simulink model "adaptive_multi_task"  (R2023b)
settings: Solver=VariableStepAuto  StartTime=0.0  StopTime=11  FixedStep=0.001
libraries: robotmaniplib x1, simulink_extras x1
settings Model: Creator=ACL_2024N02  LastModifiedBy=ACL_2024N02

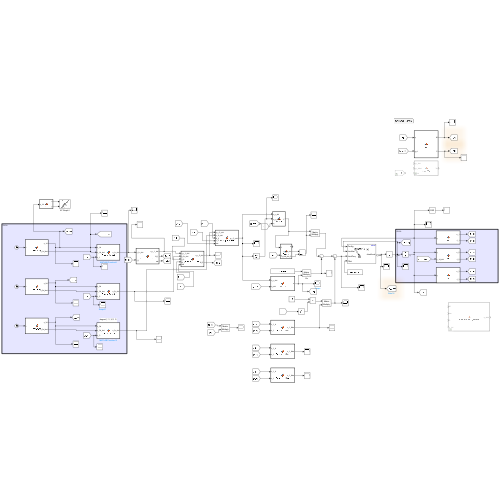
[thumbnail: Simulink's stored preview of the top-level diagram]
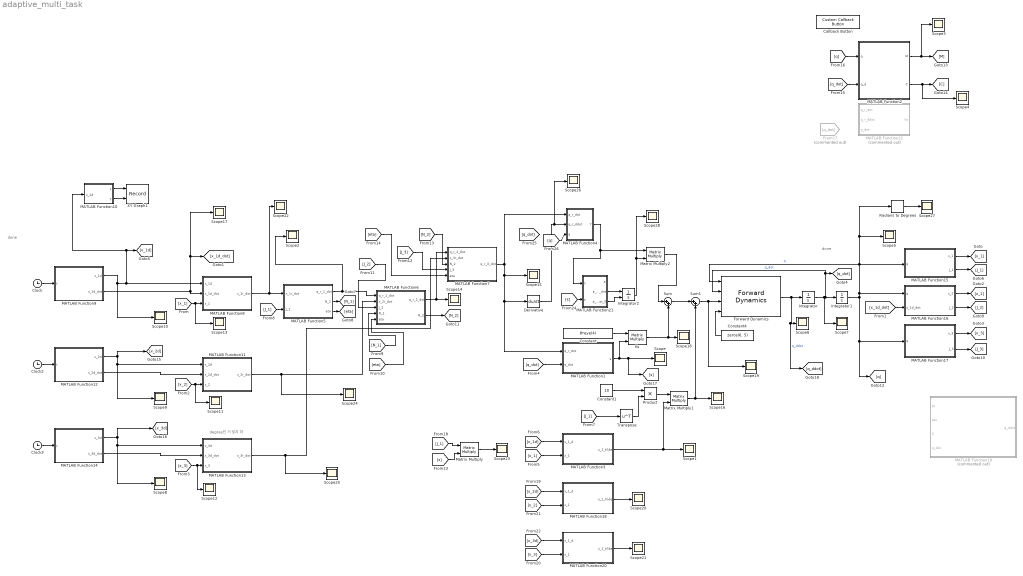
== system adaptive_multi_task ==
  note: done
  note: degree인 거 잊지 마
  note: done
  Callback Button : CustomCallbackButton  Configuration="{\"components\":[{\"name\":\"BackgroundImageComponent\",\"settings\":{\"image\":{\"size\":[0,0],\"src\":\"default\",\"srcOrientation\":\"Right\"},\"position\":[0,0,1,1]}},{\"name\":\"ButtonStateComponent\",\"settings\":{\"buttonType\":\"momentary\",\"clickFcn\":\"%% Robot kinematics setup \\n\\nrobot = rigidBodyTree;\\n\\n% 링크 생성\\nlink0 = rigidBody('link0');\\nlink1 = rigidBody('link1');\\nlink2 = rigidBody('link2');\\nlink3 = rigidBody('link3');\\nlink4 = rigidBody('link4');\\n\\n% 조인트 생성\\njoint0 = rigidBodyJoint('joint0','revolute');\\njoint1 = rigidBodyJoint('joint1','revolute');\\njoint2 = rigidBodyJoint('joint2','revolute');\\njoint3 = rigidBodyJoint('joint3','revolute');\\njoint4 = rigidBodyJoint('joint4','fixed');\\n\\n% 링크 길이 정의\\nlink_lengths = [0.5 0.4 0.35 0.2];\\n\\n% 각 조인트의 상대 위치 지정 (이전 링크 기준 x축 방향으로 이동)\\nsetFixedTransform(joint0, trvec2tform([0, 0, 0]));            % base 위치\\nsetFixedTransform(joint1, trvec2tform([link_lengths(1), 0, 0]));\\nsetFixedTransform(joint2, trvec2tform([link_lengths(2), 0, 0]));\\nsetFixedTransform(joint3, trvec2tform([link_lengths(3), 0, 0]));\\nsetFixedTransform(joint4, trvec2tform([link_lengths(4), 0, 0]));\\n\\n% 조인트를 링크에 부착\\nlink0.Joint = joint0;\\nlink1.Joint = joint1;\\nlink2.Joint = joint2;\\nlink3.Joint = joint3;\\nlink4.Joint = joint4;   \\n\\n% 링크를 트리에 추가\\naddBody(robot, link0, 'base');\\naddBody(robot, link1, 'link0');\\naddBody(robot, link2, 'link1');\\naddBody(robot, link3, 'link2');\\naddBody(robot, link4, 'link3');\\n\\n% 로봇 정보 확인\\nshowdetails(robot);\",\"onValue\":1,\"position\":[0,0,1,1],\"pressDelay\":\"500\",\"pressFcn\":\"\",\"repeatInterval\":\"0\",\"states\":[{\"horizontalAlignment\":\"center\",\"image\":{\"position\":[0,0,1,1],\"size\":[1,1],\"src\":\"default\",\"srcOrientation\":\"Right\"},\"label\":{\"color\":[0.01176470588,0.01176470588,0.01176470588,1],\"icon\":{\"size\":[0,0],\"src\":\"default\",\"srcOrientation\":\"Right\"},\"iconPlacement\":\"left\",\"opacity\":1,\"show\":true,\"text\":{\"content\":\"Callback Button\",\"font\":\"Helvetica\",\"fontSize\":9.600000000000001}},\"labelOffset\":[0,0],\"verticalAlignment\":\"middle\"},{\"horizontalAlignment\":\"center\",\"image\":{\"position\":[0,0,1,1],\"size\":[1,1],\"src\":\"default\",\"srcOrientation\":\"Right\"},\"label\":{\"color\":[0.01176470588,0.01176470588,0.01176470588,1],\"icon\":{\"size\":[0,0],\"src\":\"default\",\"srcOrientation\":\"Right\"},\"iconPlacement\":\"left\",\"opacity\":1,\"show\":true,\"text\":{\"content\":\"Callback Button\",\"font\":\"Helvetica\",\"fontSize\":9.600000000000001}},\"labelOffset\":[0,0],\"verticalAlignment\":\"middle\"},{\"horizontalAlignment\":\"center\",\"image\":{\"position\":[0,0,1,1],\"size\":[1,1],\"src\":\"default\",\"srcOrientation\":\"Right\"},\"label\":{\"color\":[0.01176470588,0.01176470588,0.01176470588,1],\"icon\":{\"size\":[0,0],\"src\":\"default\",\"srcOrientation\":\"Right\"},\"iconPlacement\":\"left\",\"opacity\":1,\"show\":true,\"text\":{\"content\":\"Callback Button\",\"font\":\"Helvetica\",\"fontSize\":9.600000000000001}},\"labelOffset\":[0,0],\"verticalAlignment\":\"middle\"},{\"horizontalAlignment\":\"center\",\"image\":{\"position\":[0,0,1,1],\"size\":[1,1],\"src\":\"default\",\"srcOrientation\":\"Right\"},\"label\":{\"color\":[0.01176470588,0.01176470588,0.01176470588,1],\"icon\":{\"size\":[0,0],\"src\":\"default\",\"srcOrientation\":\"Right\"},\"iconPlacement\":\"left\",\"opacity\":1,\"show\":true,\"text\":{\"content\":\"Callback Button\",\"font\":\"Helvetica\",\"fontSize\":9.600000000000001}},\"labelOffset\":[0,0],\"verticalAlignment\":\"middle\"}]}},{\"name\":\"ForegroundImageComponent\",\"settings\":{\"image\":{\"size\":[0,0],\"src\":\"default\",\"srcOrientation\":\"Right\"},\"isForeground\":1,\"position\":[0,0,1,1]}}],\"settings\":{\"BindingType\":\"standalone\",\"backgroundColor\":[244,244,244,1],\"backgroundOffset\":0.2,\"backgroundOpacity\":1,\"fixedAspectRatio\":\"off\",\"foregroundColor\":[0.01176470588,0.01176470588,0.01176470588,1],\"migratedFromLegacy\":true,\"useBackgroundColor\":true,\"variant\":\"callback\",\"version\":\"R2023a\"},\"type\":\"Button\"}"  CustomBackgroundColor="{\"color\":[0.9568627451,0.9568627451,0.9568627451],\"show\":true}"
  Clock : Clock
  Clock2 : Clock
  Clock3 : Clock
  Constant : Constant  Value=8*eye(4)
  Constant1 : Constant  Value=10
  Constant4 : Constant  Value=zeros(6, 5)
  Derivative : Derivative
  Forward Dynamics : robotmaniplib/Forward Dynamics  RigidBodyTree=robot  SimulateUsing=Code generation
  From17 : From  Commented=on  GotoTag=q_dot
  Integrator : Integrator  UpperSaturationLimit=pi  LowerSaturationLimit=-pi
  Integrator1 : Integrator  InitialCondition=[0.8727; 1.7; -1.6; 0.85]  UpperSaturationLimit=pi  LowerSaturationLimit=-pi
  Integrator2 : Integrator  InitialConditionSource=external
  Ks : Product  Multiplication=Matrix(*)
  MATLAB Function1 : MATLAB Function  TreatAsAtomicUnit=on
  MATLAB Function10 : MATLAB Function  TreatAsAtomicUnit=on
  MATLAB Function11 : MATLAB Function  TreatAsAtomicUnit=on
  MATLAB Function12 : MATLAB Function  TreatAsAtomicUnit=on
  MATLAB Function13 : MATLAB Function  TreatAsAtomicUnit=on
  MATLAB Function14 : MATLAB Function  TreatAsAtomicUnit=on
  MATLAB Function15 : MATLAB Function  TreatAsAtomicUnit=on
  MATLAB Function16 : MATLAB Function  TreatAsAtomicUnit=on
  MATLAB Function17 : MATLAB Function  TreatAsAtomicUnit=on
  MATLAB Function18 : MATLAB Function  TreatAsAtomicUnit=on
  MATLAB Function19 : MATLAB Function  Commented=on  TreatAsAtomicUnit=on
  MATLAB Function2 : MATLAB Function  TreatAsAtomicUnit=on
  MATLAB Function20 : MATLAB Function  TreatAsAtomicUnit=on
  MATLAB Function21 : MATLAB Function  TreatAsAtomicUnit=on
  MATLAB Function22 : MATLAB Function  Commented=on  TreatAsAtomicUnit=on
  MATLAB Function3 : MATLAB Function  TreatAsAtomicUnit=on
  MATLAB Function4 : MATLAB Function  TreatAsAtomicUnit=on
  MATLAB Function5 : MATLAB Function  TreatAsAtomicUnit=on
  MATLAB Function6 : MATLAB Function  TreatAsAtomicUnit=on
  MATLAB Function7 : MATLAB Function  TreatAsAtomicUnit=on
  MATLAB Function8 : MATLAB Function  TreatAsAtomicUnit=on
  MATLAB Function9 : MATLAB Function  TreatAsAtomicUnit=on
  Matrix Multiply : Product  Multiplication=Matrix(*)
  Matrix Multiply1 : Product  Multiplication=Matrix(*)
  Matrix Multiply2 : Product  Multiplication=Matrix(*)
  Product : Product
  Radians to Degrees : simulink_extras/Transformations/Radians to Degrees
  Scope{,1..28} (29 alike) : Scope
  Sum : Sum  Inputs=|++
  Sum1 : Sum  Inputs=|++
  Transpose : Math  Operator=transpose
  XY Graph1 : Record  FileSettingsInternal="{\"entries\":[{\"content\":{\"excelSettings\":{\"content\":{},\"type\":\"Streamout.ExcelSettings\"}},\"type\":\"Streamout.FileSettingStorage\",\"uuid\":\"\"}],\"packageUris\":[\"http:\\/\\/schema.mathworks.com\\/mf0\\/streamout_blocks\\/R2020a\"],\"version\":\"1.0\"}"  Layout=[1 1]  SignalsInternal="{\"entries\":[{\"content\":{\"signals\":[{\"content\":{\"blockPath\":[],\"dimensions\":[1],\"domain\":\"\",\"lineColor\":\"#a2142f\",\"plots\":[ 1 ],\"port\":1,\"sid\":[\"\"],\"signalID\":1,\"signalName\":\"MATLAB Function10:1\"},\"type\":\"RecordBlkView.Signal\",\"uuid\":\"\"},{\"content\":{\"blockPath\":[],\"dimensions\":[1],\"domain\":\"\",\"lineColor\":\"#139fff\",\"plots\":[ 1 ],\"port\":2,\"sid\":[\"\"],\"signalID\":2,\"signalName\":\"MATLAB Function10:2\"},\"type\":\"RecordBlkView.Signal\",\"uuid\":\"\"}]},\"type\":\"RecordBlkView.InputSignals\",\"uuid\":\"\"}],\"packageUris\":[\"http:\\/\\/schema.mathworks.com\\/mf0\\/streamout_blocks\\/R2020a\"],\"version\":\"1.0\"}"  VisualizationBindings="{\"xyplotplugin\":{\"info\":[{\"series\":[{\"bindingParametersList\":[{\"parameter\":\"X-Axis\",\"signalID\":1,\"signalName\":\"MATLAB Function10:1\"},{\"parameter\":\"Y-Axis\",\"signalID\":2,\"signalName\":\"MATLAB Function10:2\"}],\"seriesID\":0}],\"subplotID\":1}]}}"  CompatibilityTag=XY
  wires:
  Constant/1 -> Ks/1
  MATLAB Function1/1(s) -> Ks/2, Scope/1, [s]
  [J_1] -> Transpose/1
  Constant1/1 -> Product/1
  Product/1 -> Matrix Multiply1/1
  MATLAB Function3/1(x_1_tilde) -> Scope1/1, Matrix Multiply1/2
  Ks/1 -> Scope18/1, Sum/2
  Sum/1 -> Sum1/1
  Matrix Multiply1/1 -> Sum1/2, Scope16/1
  Sum1/1 -> Scope19/1, Forward Dynamics/3
  Constant4/1 -> Forward Dynamics/4
  Forward Dynamics/1 -> [q_ddot], Scope6/1, Integrator/1  "q_ddot"
  Integrator/1 -> Integrator1/1, Forward Dynamics/2, [q_dot], Scope7/1  "q_dot"
  Integrator1/1 -> Forward Dynamics/1, Radians to Degrees/1, Scope5/1, MATLAB Function15/1(q), MATLAB Function16/1(q), [q], MATLAB Function17/1(q)  "q"
  MATLAB Function5/1(q_r_1_dot) -> Scope2/1, MATLAB Function6/1(q_r_1_dot)
  MATLAB Function6/1(q_r_2_dot) -> Scope14/1, MATLAB Function7/1(q_r_2_dot)
  MATLAB Function7/1(q_r_3_dot) -> Derivative/1, MATLAB Function1/1(q_r_dot), Scope15/1, MATLAB Function4/1(q_r_dot)
  MATLAB Function9/1(x_1d) -> Scope10/1, MATLAB Function8/1(x_1d), MATLAB Function10/1(x_1d), [x_1d]
  MATLAB Function9/2(x_1d_dot) -> MATLAB Function8/2(x_1d_dot), [x_1d_dot], Scope17/1
  Clock/1 -> MATLAB Function9/1(t)
  MATLAB Function8/1(x_1r_dot) -> Scope22/1, MATLAB Function5/1(x_1r_dot)
  MATLAB Function12/1(x_2d) -> Scope9/1, MATLAB Function11/1(x_2d), [x_2d]
  Clock2/1 -> MATLAB Function12/1(t)
  MATLAB Function12/2(x_2d_dot) -> MATLAB Function11/2(x_2d_dot)
  Clock3/1 -> MATLAB Function14/1(t)
  MATLAB Function14/1(x_3d) -> Scope8/1, MATLAB Function13/1(x_3d), [x_3d]
  MATLAB Function15/1(x_1) -> [x_1]
  [x_1] -> Scope13/1, MATLAB Function8/3(x_1)
  [x_1d_dot] -> MATLAB Function16/2(x_1d_dot)
  MATLAB Function16/1(x_2) -> [x_2]
  [x_2] -> Scope11/1, MATLAB Function11/3(x_2)
  MATLAB Function17/1(x_3) -> [x_3]
  [x_3] -> Scope12/1, MATLAB Function13/3(x_3)
  MATLAB Function11/1(x_2r_dot) -> Scope24/1, MATLAB Function6/2(x_2r_dot)
  MATLAB Function13/1(x_3r_dot) -> Scope25/1, MATLAB Function7/2(x_3r_dot)
  Derivative/1 -> Scope26/1, MATLAB Function4/2(q_r_ddot)
  [q_dot] -> MATLAB Function1/2(q_dot)
  [x_1] -> MATLAB Function3/2(x_1)
  [x_1d] -> MATLAB Function3/1(x_1_d)
  MATLAB Function15/2(J_1) -> [J_1]
  [J_1] -> MATLAB Function5/2(J_1)
  MATLAB Function5/2(N_1) -> [N_1]
  [N_1] -> MATLAB Function6/4(N_1)
  MATLAB Function5/3(eta) -> [eta]
  [eta] -> MATLAB Function6/5(eta)
  MATLAB Function16/2(J_2) -> [J_2]
  [J_2] -> MATLAB Function6/3(J_2)
  MATLAB Function17/2(J_3) -> [J_3]
  MATLAB Function6/2(N_2) -> [N_2]
  [N_2] -> MATLAB Function7/3(N_2)
  [J_3] -> MATLAB Function7/4(J_3)
  [eta] -> MATLAB Function7/5(eta)
  Transpose/1 -> Product/2
  [q_dot] -> MATLAB Function2/2(q_d)
  [q] -> MATLAB Function2/1(q)
  MATLAB Function2/1(M) -> Scope3/1, [M]
  MATLAB Function2/2(C) -> Scope4/1, [C]
  MATLAB Function10/1(x) -> XY Graph1/1
  MATLAB Function10/2(y) -> XY Graph1/2
  [x_2] -> MATLAB Function18/2(x_1)
  [x_2d] -> MATLAB Function18/1(x_1_d)
  [x_3] -> MATLAB Function20/2(x_1)
  [x_3d] -> MATLAB Function20/1(x_1_d)
  MATLAB Function18/1(x_1_tilde) -> Scope20/1
  MATLAB Function20/1(x_1_tilde) -> Scope21/1
  MATLAB Function14/2(x_3d_dot) -> MATLAB Function13/2(x_3d_dot)
  [J_1] -> Matrix Multiply/1
  [s] -> Matrix Multiply/2
  Matrix Multiply/1 -> Scope23/1
  MATLAB Function4/1(Y) -> MATLAB Function21/1(Y), Matrix Multiply2/1
  [s] -> MATLAB Function21/2(s)
  MATLAB Function21/2(a_hat_dot) -> Integrator2/1
  MATLAB Function21/3(a_hat_dot_0) -> Integrator2/2
  Matrix Multiply2/1 -> Sum/1
  Radians to Degrees/1 -> Scope27/1
  [q] -> MATLAB Function4/3(q)
  Integrator2/1 -> Scope28/1, Matrix Multiply2/2

== matlab function adaptive_multi_task/MATLAB Function11 ==
  data: x_2r_dot output; x_2d input; x_2d_dot input; x_2 input
function x_2r_dot = func_x_2r_dot(x_2d, x_2d_dot, x_2)

Gamma_2 = 4*eye(1)

x_2r_dot = x_2d_dot + Gamma_2*(x_2d - x_2)

== matlab function adaptive_multi_task/MATLAB Function12 ==
  data: x_2d output; t input; x_2d_dot output
function [x_2d, x_2d_dot] = func_x_2d(t)

x_2d = atan2(-sin(0.25*t),cos(0.25*t))+pi/2
x_2d_dot = -0.25

== matlab function adaptive_multi_task/MATLAB Function13 ==
  data: x_3r_dot output; x_3d input; x_3d_dot input; x_3 input
function x_3r_dot = func_x_3r_dot(x_3d, x_3d_dot, x_3)

Gamma_3 = 4*eye(1)

x_3r_dot = x_3d_dot + Gamma_3*(x_3d - x_3)

== matlab function adaptive_multi_task/MATLAB Function14 ==
  data: x_3d output; t input; x_3d_dot output
function [x_3d, x_3d_dot] = func_x_3d(t)

x_3d = deg2rad(35) % degree
x_3d_dot = 0

== matlab function adaptive_multi_task/MATLAB Function15 ==
  data: q input; x_1 output; J_1 output
function [x_1, J_1] = fcn(q)
% current end-effector position

l1 = 0.5 % meters
l2 = 0.4
l3 = 0.35
l4 = 0.2

q1 = q(1)
q2 = q(2)
q3 = q(3)
q4 = q(4)

x_1 = [l1*cos(q1)+l2*cos(q1+q2)+l3*cos(q1+q2+q3)+l4*cos(q1+q2+q3+q4); ...
    l1*sin(q1)+l2*sin(q1+q2)+l3*sin(q1+q2+q3)+l4*sin(q1+q2+q3+q4)]

J_1 = [-l1*sin(q1), -l2*sin(q1+q2), -l3*sin(q1+q2+q3), -l4*sin(q1+q2+q3+q4); ...
    l1*cos(q1),  l2*cos(q1+q2),  l3*cos(q1+q2+q3),  l4*cos(q1+q2+q3+q4)]

== matlab function adaptive_multi_task/MATLAB Function16 ==
  data: q input; x_2 output; x_1d_dot input; J_2 output
function [x_2, J_2] = fcn(q, x_1d_dot)

q1 = q(1)
q2 = q(2)
q3 = q(3)
q4 = q(4)

theta4 = q1+q2+q3+q4
direction4 = [cos(theta4); sin(theta4)]

x_2 = theta4


J_2 = [1 1 1 1]

== matlab function adaptive_multi_task/MATLAB Function1 ==
  data: s output; q_r_dot input; q_dot input
function s = func_s(q_r_dot, q_dot)

% equation 15
s = q_r_dot - q_dot

== matlab function adaptive_multi_task/MATLAB Function17 ==
  data: q input; x_3 output; J_3 output
function [x_3, J_3] = fcn(q)

x_3 = q(1)
J_3 = [1, 0, 0, 0]

== matlab function adaptive_multi_task/MATLAB Function18 ==
  data: x_1_tilde output; x_1_d input; x_1 input
function x_1_tilde = func_x_1_tilde(x_1_d, x_1)

x_1_tilde = x_1_d - x_1

== matlab function adaptive_multi_task/MATLAB Function19 ==
  data: M input; q_ddot output; tau input; C input; q_dot input
function q_ddot = func_forwardDynamics(M, tau, C, q_dot)

q_ddot = pinv(M) * (tau - C*q_dot)

== matlab function adaptive_multi_task/MATLAB Function20 ==
  data: x_1_tilde output; x_1_d input; x_1 input
function x_1_tilde = func_x_1_tilde(x_1_d, x_1)

x_1_tilde = x_1_d - x_1

== matlab function adaptive_multi_task/MATLAB Function21 ==
  data: a output; Y input; s input; a_hat_dot output; a_hat_dot_0 output
function [a, a_hat_dot, a_hat_dot_0] = func_a(Y, s)

% equation 22
% M = robot.massMatrix 
% C = diag([1.7, 1.6, 1.5, 1.4])
l1=0.5;l2=0.4;l3=0.35;l4=0.2;
m1=1.4;m2=1.3;m3=1.2;m4=1.1;
I1=0.5;I2=0.45;I3=0.4;I4=0.3;
c1=1.7;c2=1.6;c3=1.5;c4=1.4;
r1=l1/2;r2=l2/2;r3=l3/2;r4=l4/2;

a = [m1*r1^2,I1,I2,I3,I4,m2,m2*r2,m2*r2^2,m3,m3*r3,m3*r3^2,m4,m4*r4,m4*r4^2,c1,c2,c3,c4]'
a_hat_dot_0 = 0.5 * a

Gamma = diag([0.1,0.2,0.2,0.2,0.2,0.2,0.2,0.1,0.2,0.2,0.1,0.2,0.2,0.1,30,30,20,10])
a_hat_dot = Gamma * transpose(Y) * s

== matlab function adaptive_multi_task/MATLAB Function22 ==
  data: q_r_dot input; Ya output; q_r_ddot input; q_dot input
function Ya = func_Ya(q_r_dot, q_r_ddot, q_dot)

% equation 22
% M = robot.massMatrix 
% C = diag([1.7, 1.6, 1.5, 1.4])
l1=0.5;l2=0.4;l3=0.35;l4=0.2;
m1=1.4;m2=1.3;m3=1.2;m4=1.1;
I1=0.5;I2=0.45;I3=0.4;I4=0.3;
c1=1.7;c2=1.6;c3=1.5;c4=1.4;
r1=l1/2;r2=l2/2;r3=l3/2;r4=l4/2;

a = [m1*r1^2,I1,I2,I3,I4,m2,m2*r2,m2*r2^2,m3,m3*r3,m3*r3^2,m4,m4*r4,m4*r4^2,c1,c2,c3,c4]
Y = [q_r_ddot,q_r_ddot,q_r_ddot,q_r_ddot,q_r_ddot, ...
    r2^2*q_r_ddot, r2*q_r_ddot, q_r_ddot, ...
    r3^2*q_r_ddot, r3*q_r_ddot, q_r_ddot, ...
    r4^2*q_r_ddot, r4*q_r_ddot, q_r_ddot, ...
    q_dot, q_dot, q_dot, q_dot]
Ya = Y*a'

== matlab function adaptive_multi_task/MATLAB Function2 ==
  data: q input; M output; q_d input; C output
function [M, C] = fcn(q, q_d)

q1 = q(1)
q2 = q(2)
q3 = q(3)
q4 = q(4)

dq1 = q_d(1)
dq2 = q_d(2)
dq3 = q_d(3)
dq4 = q_d(4)

M = [ (11*cos(q2 + q3 + q4))/200 + (161*cos(q2 + q3))/800 + (11*cos(q3 + q4))/250 + (9*cos(q2))/25 + (161*cos(q3))/1000 + (77*cos(q4))/2000 + 35007/16000, (11*cos(q2 + q3 + q4))/400 + (161*cos(q2 + q3))/1600 + (11*cos(q3 + q4))/250 + (9*cos(q2))/50 + (161*cos(q3))/1000 + (77*cos(q4))/2000 + 22007/16000, (11*cos(q2 + q3 + q4))/400 + (161*cos(q2 + q3))/1600 + (11*cos(q3 + q4))/500 + (161*cos(q3))/2000 + (77*cos(q4))/2000 + 12503/16000, (11*cos(q2 + q3 + q4))/400 + (11*cos(q3 + q4))/500 + (77*cos(q4))/4000 + 311/1000; ...
    (11*cos(q2 + q3 + q4))/400 + (161*cos(q2 + q3))/1600 + (11*cos(q3 + q4))/250 + (9*cos(q2))/50 + (161*cos(q3))/1000 + (77*cos(q4))/2000 + 22007/16000,                                                                         (11*cos(q3 + q4))/250 + (161*cos(q3))/1000 + (77*cos(q4))/2000 + 22007/16000,                                                        (11*cos(q3 + q4))/500 + (161*cos(q3))/2000 + (77*cos(q4))/2000 + 12503/16000,                              (11*cos(q3 + q4))/500 + (77*cos(q4))/4000 + 311/1000; ...
    (11*cos(q2 + q3 + q4))/400 + (161*cos(q2 + q3))/1600 + (11*cos(q3 + q4))/500 + (161*cos(q3))/2000 + (77*cos(q4))/2000 + 12503/16000,                                                                         (11*cos(q3 + q4))/500 + (161*cos(q3))/2000 + (77*cos(q4))/2000 + 12503/16000,                                                                                                     (77*cos(q4))/2000 + 12503/16000,                                                      (77*cos(q4))/4000 + 311/1000; ...
    (11*cos(q2 + q3 + q4))/400 + (11*cos(q3 + q4))/500 + (77*cos(q4))/4000 + 311/1000,                                                                                                 (11*cos(q3 + q4))/500 + (77*cos(q4))/4000 + 311/1000,                                                                                                        (77*cos(q4))/4000 + 311/1000,                                                                          311/1000]
 

C = [- dq2*((11*sin(q2 + q3 + q4))/400 + (161*sin(q2 + q3))/1600 + (9*sin(q2))/50) - dq4*((11*sin(q2 + q3 + q4))/400 + (11*sin(q3 + q4))/500 + (77*sin(q4))/4000) - dq3*((11*sin(q2 + q3 + q4))/400 + (161*sin(q2 + q3))/1600 + (11*sin(q3 + q4))/500 + (161*sin(q3))/2000), - dq1*((11*sin(q2 + q3 + q4))/400 + (161*sin(q2 + q3))/1600 + (9*sin(q2))/50) - dq2*((11*sin(q2 + q3 + q4))/400 + (161*sin(q2 + q3))/1600 + (9*sin(q2))/50) - dq4*((11*sin(q2 + q3 + q4))/400 + (11*sin(q3 + q4))/500 + (77*sin(q4))/4000) - dq3*((11*sin(q2 + q3 + q4))/400 + (161*sin(q2 + q3))/1600 + (11*sin(q3 + q4))/500 + (161*sin(q3))/2000), - dq4*((11*sin(q2 + q3 + q4))/400 + (11*sin(q3 + q4))/500 + (77*sin(q4))/4000) - dq1*((11*sin(q2 + q3 + q4))/400 + (161*sin(q2 + q3))/1600 + (11*sin(q3 + q4))/500 + (161*sin(q3))/2000) - dq2*((11*sin(q2 + q3 + q4))/400 + (161*sin(q2 + q3))/1600 + (11*sin(q3 + q4))/500 + (161*sin(q3))/2000) - dq3*((11*sin(q2 + q3 + q4))/400 + (161*sin(q2 + q3))/1600 + (11*sin(q3 + q4))/500 + (161*sin(q3))/2000), -(11*(10*sin(q2 + q3 + q4) + 8*sin(q3 + q4) + 7*sin(q4))*(dq1 + dq2 + dq3 + dq4))/4000; ...
    dq1*((11*sin(q2 + q3 + q4))/400 + (161*sin(q2 + q3))/1600 + (9*sin(q2))/50) - dq3*((11*sin(q3 + q4))/500 + (161*sin(q3))/2000) - dq4*((11*sin(q3 + q4))/500 + (77*sin(q4))/4000),                                                                                                                                                                                                                                                 - dq3*((11*sin(q3 + q4))/500 + (161*sin(q3))/2000) - dq4*((11*sin(q3 + q4))/500 + (77*sin(q4))/4000),                                                                                                                                                                                                   - dq1*((11*sin(q3 + q4))/500 + (161*sin(q3))/2000) - dq2*((11*sin(q3 + q4))/500 + (161*sin(q3))/2000) - dq3*((11*sin(q3 + q4))/500 + (161*sin(q3))/2000) - dq4*((11*sin(q3 + q4))/500 + (77*sin(q4))/4000),                        -(11*(8*sin(q3 + q4) + 7*sin(q4))*(dq1 + dq2 + dq3 + dq4))/4000; ...
    dq1*((11*sin(q2 + q3 + q4))/400 + (161*sin(q2 + q3))/1600 + (11*sin(q3 + q4))/500 + (161*sin(q3))/2000) + dq2*((11*sin(q3 + q4))/500 + (161*sin(q3))/2000) - (77*dq4*sin(q4))/4000,                                                                                                                                                                                                                          dq1*((11*sin(q3 + q4))/500 + (161*sin(q3))/2000) + dq2*((11*sin(q3 + q4))/500 + (161*sin(q3))/2000) - (77*dq4*sin(q4))/4000,                                                                                                                                                                                                                                                                                                                                                                                       -(77*dq4*sin(q4))/4000,                                             -(77*sin(q4)*(dq1 + dq2 + dq3 + dq4))/4000; ...
    dq1*((11*sin(q2 + q3 + q4))/400 + (11*sin(q3 + q4))/500 + (77*sin(q4))/4000) + dq2*((11*sin(q3 + q4))/500 + (77*sin(q4))/4000) + (77*dq3*sin(q4))/4000,                                                                                                                                                                                                                            dq1*((11*sin(q3 + q4))/500 + (77*sin(q4))/4000) + dq2*((11*sin(q3 + q4))/500 + (77*sin(q4))/4000) + (77*dq3*sin(q4))/4000,                                                                                                                                                                                                                                                                                                                                                                          (77*sin(q4)*(dq1 + dq2 + dq3))/4000,                                                                                      0]
 

end

== matlab function adaptive_multi_task/MATLAB Function3 ==
  data: x_1_tilde output; x_1_d input; x_1 input
function x_1_tilde = func_x_1_tilde(x_1_d, x_1)

x_1_tilde = x_1_d - x_1

== matlab function adaptive_multi_task/MATLAB Function4 ==
  data: q_r_dot input; Y output; q_r_ddot input; q input
function Y = func_Y(q_r_dot, q_r_ddot, q)

l1=0.5;l2=0.4;l3=0.35;l4=0.2;
m1=1.4;m2=1.3;m3=1.2;m4=1.1;
I1=0.5;I2=0.45;I3=0.4;I4=0.3;
c1=1.7;c2=1.6;c3=1.5;c4=1.4;
r1=l1/2;r2=l2/2;r3=l3/2;r4=l4/2;

qr1_dot = q_r_dot(1)
qr2_dot = q_r_dot(2)
qr3_dot = q_r_dot(3)
qr4_dot = q_r_dot(4)

qr1_ddot = q_r_ddot(1)
qr2_ddot = q_r_ddot(2)
qr3_ddot = q_r_ddot(3)
qr4_ddot = q_r_ddot(4)

qq1 = q(1)
qq2 = q(2)
qq3 = q(3)
qq4 = q(4)

% Y = [q_r_ddot,q_r_ddot,q_r_ddot,q_r_ddot,q_r_ddot, ...
%     r2^2*q_r_ddot, r2*q_r_ddot, q_r_ddot, ...
%     r3^2*q_r_ddot, r3*q_r_ddot, q_r_ddot, ...
%     r4^2*q_r_ddot, r4*q_r_ddot, q_r_ddot, ...
%     q_dot, q_dot, q_dot, q_dot]


 
Y = [qr1_ddot, qr1_ddot, qr1_ddot + qr2_ddot, qr1_ddot + qr2_ddot + qr3_ddot, qr1_ddot + qr2_ddot + qr3_ddot + qr4_ddot, l1^2*qr1_ddot, qr1_ddot*r2 + qr2_ddot*r2 + 2*l1*qr1_ddot*cos(qq2) + l1*qr2_ddot*cos(qq2) + 2*l1*qr1_dot*sin(qq2) - 2*l1*qr2_dot*sin(qq2), 0, l1^2*qr1_ddot + l2^2*qr1_ddot + l2^2*qr2_ddot + 2*l1*l2*qr1_ddot*cos(qq2) + l1*l2*qr2_ddot*cos(qq2) + 2*l1*l2*qr1_dot*sin(qq2) - 2*l1*l2*qr2_dot*sin(qq2), qr1_ddot*r3 + qr2_ddot*r3 + qr3_ddot*r3 + 2*l2*qr1_ddot*cos(qq3) + 2*l2*qr2_ddot*cos(qq3) + l2*qr3_ddot*cos(qq3) + 2*l2*qr1_dot*sin(qq3) + 2*l2*qr2_dot*sin(qq3) - 4*l2*qr3_dot*sin(qq3) + 2*l1*qr1_ddot*cos(qq2 + qq3) + l1*qr2_ddot*cos(qq2 + qq3) + l1*qr3_ddot*cos(qq2 + qq3) + 4*l1*qr1_dot*sin(qq2 + qq3) - 2*l1*qr2_dot*sin(qq2 + qq3) - 2*l1*qr3_dot*sin(qq2 + qq3), 0, l1^2*qr1_ddot + l2^2*qr1_ddot + l2^2*qr2_ddot + (l3^2*qr1_ddot)/2 + (l3^2*qr2_ddot)/2 + (l3^2*qr3_ddot)/2 + (qr1_ddot*r3^2)/2 + (qr2_ddot*r3^2)/2 + (qr3_ddot*r3^2)/2 - (l3^2*qr1_ddot*cos(2*qq1 + 2*qq2 + 2*qq3))/2 - (l3^2*qr2_ddot*cos(2*qq1 + 2*qq2 + 2*qq3))/2 - (l3^2*qr3_ddot*cos(2*qq1 + 2*qq2 + 2*qq3))/2 + (qr1_ddot*r3^2*cos(2*qq1 + 2*qq2 + 2*qq3))/2 + (qr2_ddot*r3^2*cos(2*qq1 + 2*qq2 + 2*qq3))/2 + (qr3_ddot*r3^2*cos(2*qq1 + 2*qq2 + 2*qq3))/2 + 3*l3^2*qr1_dot*sin(2*qq1 + 2*qq2 + 2*qq3) + 3*l3^2*qr2_dot*sin(2*qq1 + 2*qq2 + 2*qq3) + 3*l3^2*qr3_dot*sin(2*qq1 + 2*qq2 + 2*qq3) - 3*qr1_dot*r3^2*sin(2*qq1 + 2*qq2 + 2*qq3) - 3*qr2_dot*r3^2*sin(2*qq1 + 2*qq2 + 2*qq3) - 3*qr3_dot*r3^2*sin(2*qq1 + 2*qq2 + 2*qq3) - l1*l3*qr1_ddot*cos(2*qq1 + qq2 + qq3) - (l1*l3*qr2_ddot*cos(2*qq1 + qq2 + qq3))/2 - (l1*l3*qr3_ddot*cos(2*qq1 + qq2 + qq3))/2 + l1*qr1_ddot*r3*cos(2*qq1 + qq2 + qq3) + (l1*qr2_ddot*r3*cos(2*qq1 + qq2 + qq3))/2 + (l1*qr3_ddot*r3*cos(2*qq1 + qq2 + qq3))/2 + 4*l1*l3*qr1_dot*sin(2*qq1 + qq2 + qq3) + l1*l3*qr2_dot*sin(2*qq1 + qq2 + qq3) + l1*l3*qr3_dot*sin(2*qq1 + qq2 + qq3) - 4*l1*qr1_dot*r3*sin(2*qq1 + qq2 + qq3) - l1*qr2_dot*r3*sin(2*qq1 + qq2 + qq3) - l1*qr3_dot*r3*sin(2*qq1 + qq2 + qq3) + l1*l3*qr1_ddot*cos(qq2 + qq3) + (l1*l3*qr2_ddot*cos(qq2 + qq3))/2 + (l1*l3*qr3_ddot*cos(qq2 + qq3))/2 + l1*qr1_ddot*r3*cos(qq2 + qq3) + (l1*qr2_ddot*r3*cos(qq2 + qq3))/2 + (l1*qr3_ddot*r3*cos(qq2 + qq3))/2 + 2*l1*l3*qr1_dot*sin(qq2 + qq3) - l1*l3*qr2_dot*sin(qq2 + qq3) - l1*l3*qr3_dot*sin(qq2 + qq3) + 2*l1*qr1_dot*r3*sin(qq2 + qq3) - l1*qr2_dot*r3*sin(qq2 + qq3) - l1*qr3_dot*r3*sin(qq2 + qq3) + 2*l1*l2*qr1_ddot*cos(qq2) + l1*l2*qr2_ddot*cos(qq2) + l2*l3*qr1_ddot*cos(qq3) + l2*l3*qr2_ddot*cos(qq3) + (l2*l3*qr3_ddot*cos(qq3))/2 - l2*l3*qr1_ddot*cos(2*qq1 + 2*qq2 + qq3) - l2*l3*qr2_ddot*cos(2*qq1 + 2*qq2 + qq3) - (l2*l3*qr3_ddot*cos(2*qq1 + 2*qq2 + qq3))/2 + l2*qr1_ddot*r3*cos(qq3) + l2*qr2_ddot*r3*cos(qq3) + (l2*qr3_ddot*r3*cos(qq3))/2 + l2*qr1_ddot*r3*cos(2*qq1 + 2*qq2 + qq3) + l2*qr2_ddot*r3*cos(2*qq1 + 2*qq2 + qq3) + (l2*qr3_ddot*r3*cos(2*qq1 + 2*qq2 + qq3))/2 + 2*l1*l2*qr1_dot*sin(qq2) - 2*l1*l2*qr2_dot*sin(qq2) + l2*l3*qr1_dot*sin(qq3) + l2*l3*qr2_dot*sin(qq3) - 2*l2*l3*qr3_dot*sin(qq3) + 5*l2*l3*qr1_dot*sin(2*qq1 + 2*qq2 + qq3) + 5*l2*l3*qr2_dot*sin(2*qq1 + 2*qq2 + qq3) + 2*l2*l3*qr3_dot*sin(2*qq1 + 2*qq2 + qq3) + l2*qr1_dot*r3*sin(qq3) + l2*qr2_dot*r3*sin(qq3) - 2*l2*qr3_dot*r3*sin(qq3) - 5*l2*qr1_dot*r3*sin(2*qq1 + 2*qq2 + qq3) - 5*l2*qr2_dot*r3*sin(2*qq1 + 2*qq2 + qq3) - 2*l2*qr3_dot*r3*sin(2*qq1 + 2*qq2 + qq3), qr1_ddot*r4 + qr2_ddot*r4 + qr3_ddot*r4 + qr4_ddot*r4 + l3*qr1_ddot*cos(qq4) + l3*qr2_ddot*cos(qq4) + l3*qr3_ddot*cos(qq4) + (l3*qr4_ddot*cos(qq4))/2 + qr1_ddot*r3*cos(qq4) + qr2_ddot*r3*cos(qq4) + qr3_ddot*r3*cos(qq4) + (qr4_ddot*r3*cos(qq4))/2 + l3*qr1_dot*sin(qq4) + l3*qr2_dot*sin(qq4) + l3*qr3_dot*sin(qq4) - 3*l3*qr4_dot*sin(qq4) + qr1_dot*r3*sin(qq4) + qr2_dot*r3*sin(qq4) + qr3_dot*r3*sin(qq4) - 3*qr4_dot*r3*sin(qq4) + 2*l1*qr1_ddot*cos(qq2 + qq3 + qq4) + l1*qr2_ddot*cos(qq2 + qq3 + qq4) + l1*qr3_ddot*cos(qq2 + qq3 + qq4) + l1*qr4_ddot*cos(qq2 + qq3 + qq4) + 6*l1*qr1_dot*sin(qq2 + qq3 + qq4) - 2*l1*qr2_dot*sin(qq2 + qq3 + qq4) - 2*l1*qr3_dot*sin(qq2 + qq3 + qq4) - 2*l1*qr4_dot*sin(qq2 + qq3 + qq4) + 2*l2*qr1_ddot*cos(qq3 + qq4) + 2*l2*qr2_ddot*cos(qq3 + qq4) + l2*qr3_ddot*cos(qq3 + qq4) + l2*qr4_ddot*cos(qq3 + qq4) - l3*qr1_ddot*cos(2*qq1 + 2*qq2 + 2*qq3 + qq4) - l3*qr2_ddot*cos(2*qq1 + 2*qq2 + 2*qq3 + qq4) - l3*qr3_ddot*cos(2*qq1 + 2*qq2 + 2*qq3 + qq4) - (l3*qr4_ddot*cos(2*qq1 + 2*qq2 + 2*qq3 + qq4))/2 + qr1_ddot*r3*cos(2*qq1 + 2*qq2 + 2*qq3 + qq4) + qr2_ddot*r3*cos(2*qq1 + 2*qq2 + 2*qq3 + qq4) + qr3_ddot*r3*cos(2*qq1 + 2*qq2 + 2*qq3 + qq4) + (qr4_ddot*r3*cos(2*qq1 + 2*qq2 + 2*qq3 + qq4))/2 + 4*l2*qr1_dot*sin(qq3 + qq4) + 4*l2*qr2_dot*sin(qq3 + qq4) - 4*l2*qr3_dot*sin(qq3 + qq4) - 4*l2*qr4_dot*sin(qq3 + qq4) + 7*l3*qr1_dot*sin(2*qq1 + 2*qq2 + 2*qq3 + qq4) + 7*l3*qr2_dot*sin(2*qq1 + 2*qq2 + 2*qq3 + qq4) + 7*l3*qr3_dot*sin(2*qq1 + 2*qq2 + 2*qq3 + qq4) + 3*l3*qr4_dot*sin(2*qq1 + 2*qq2 + 2*qq3 + qq4) - 7*qr1_dot*r3*sin(2*qq1 + 2*qq2 + 2*qq3 + qq4) - 7*qr2_dot*r3*sin(2*qq1 + 2*qq2 + 2*qq3 + qq4) - 7*qr3_dot*r3*sin(2*qq1 + 2*qq2 + 2*qq3 + qq4) - 3*qr4_dot*r3*sin(2*qq1 + 2*qq2 + 2*qq3 + qq4), 0, 0, 0, 0, 0; ...
    0,        0, qr1_ddot + qr2_ddot, qr1_ddot + qr2_ddot + qr3_ddot, qr1_ddot + qr2_ddot + qr3_ddot + qr4_ddot,             0,                          qr1_ddot*r2 + qr2_ddot*r2 + l1*qr1_ddot*cos(qq2) - 2*l1*qr1_dot*sin(qq2) - 2*l1*qr2_dot*sin(qq2), 0,                                                     l2*(l2*qr1_ddot + l2*qr2_ddot + l1*qr1_ddot*cos(qq2) - 2*l1*qr1_dot*sin(qq2) - 2*l1*qr2_dot*sin(qq2)),                                                             qr1_ddot*r3 + qr2_ddot*r3 + qr3_ddot*r3 + 2*l2*qr1_ddot*cos(qq3) + 2*l2*qr2_ddot*cos(qq3) + l2*qr3_ddot*cos(qq3) + 2*l2*qr1_dot*sin(qq3) + 2*l2*qr2_dot*sin(qq3) - 4*l2*qr3_dot*sin(qq3) + l1*qr1_ddot*cos(qq2 + qq3) - 2*l1*qr1_dot*sin(qq2 + qq3) - 2*l1*qr2_dot*sin(qq2 + qq3) - 2*l1*qr3_dot*sin(qq2 + qq3), 0,                                                                                                                                                                                                                                                                                                                                                                     l2^2*qr1_ddot + l2^2*qr2_ddot + (l3^2*qr1_ddot)/2 + (l3^2*qr2_ddot)/2 + (l3^2*qr3_ddot)/2 + (qr1_ddot*r3^2)/2 + (qr2_ddot*r3^2)/2 + (qr3_ddot*r3^2)/2 - (l3^2*qr1_ddot*cos(2*qq1 + 2*qq2 + 2*qq3))/2 - (l3^2*qr2_ddot*cos(2*qq1 + 2*qq2 + 2*qq3))/2 - (l3^2*qr3_ddot*cos(2*qq1 + 2*qq2 + 2*qq3))/2 + (qr1_ddot*r3^2*cos(2*qq1 + 2*qq2 + 2*qq3))/2 + (qr2_ddot*r3^2*cos(2*qq1 + 2*qq2 + 2*qq3))/2 + (qr3_ddot*r3^2*cos(2*qq1 + 2*qq2 + 2*qq3))/2 + 3*l3^2*qr1_dot*sin(2*qq1 + 2*qq2 + 2*qq3) + 3*l3^2*qr2_dot*sin(2*qq1 + 2*qq2 + 2*qq3) + 3*l3^2*qr3_dot*sin(2*qq1 + 2*qq2 + 2*qq3) - 3*qr1_dot*r3^2*sin(2*qq1 + 2*qq2 + 2*qq3) - 3*qr2_dot*r3^2*sin(2*qq1 + 2*qq2 + 2*qq3) - 3*qr3_dot*r3^2*sin(2*qq1 + 2*qq2 + 2*qq3) - (l1*l3*qr1_ddot*cos(2*qq1 + qq2 + qq3))/2 + (l1*qr1_ddot*r3*cos(2*qq1 + qq2 + qq3))/2 + l1*l3*qr1_dot*sin(2*qq1 + qq2 + qq3) + l1*l3*qr2_dot*sin(2*qq1 + qq2 + qq3) + l1*l3*qr3_dot*sin(2*qq1 + qq2 + qq3) - l1*qr1_dot*r3*sin(2*qq1 + qq2 + qq3) - l1*qr2_dot*r3*sin(2*qq1 + qq2 + qq3) - l1*qr3_dot*r3*sin(2*qq1 + qq2 + qq3) + (l1*l3*qr1_ddot*cos(qq2 + qq3))/2 + (l1*qr1_ddot*r3*cos(qq2 + qq3))/2 - l1*l3*qr1_dot*sin(qq2 + qq3) - l1*l3*qr2_dot*sin(qq2 + qq3) - l1*l3*qr3_dot*sin(qq2 + qq3) - l1*qr1_dot*r3*sin(qq2 + qq3) - l1*qr2_dot*r3*sin(qq2 + qq3) - l1*qr3_dot*r3*sin(qq2 + qq3) + l1*l2*qr1_ddot*cos(qq2) + l2*l3*qr1_ddot*cos(qq3) + l2*l3*qr2_ddot*cos(qq3) + (l2*l3*qr3_ddot*cos(qq3))/2 - l2*l3*qr1_ddot*cos(2*qq1 + 2*qq2 + qq3) - l2*l3*qr2_ddot*cos(2*qq1 + 2*qq2 + qq3) - (l2*l3*qr3_ddot*cos(2*qq1 + 2*qq2 + qq3))/2 + l2*qr1_ddot*r3*cos(qq3) + l2*qr2_ddot*r3*cos(qq3) + (l2*qr3_ddot*r3*cos(qq3))/2 + l2*qr1_ddot*r3*cos(2*qq1 + 2*qq2 + qq3) + l2*qr2_ddot*r3*cos(2*qq1 + 2*qq2 + qq3) + (l2*qr3_ddot*r3*cos(2*qq1 + 2*qq2 + qq3))/2 - 2*l1*l2*qr1_dot*sin(qq2) - 2*l1*l2*qr2_dot*sin(qq2) + l2*l3*qr1_dot*sin(qq3) + l2*l3*qr2_dot*sin(qq3) - 2*l2*l3*qr3_dot*sin(qq3) + 5*l2*l3*qr1_dot*sin(2*qq1 + 2*qq2 + qq3) + 5*l2*l3*qr2_dot*sin(2*qq1 + 2*qq2 + qq3) + 2*l2*l3*qr3_dot*sin(2*qq1 + 2*qq2 + qq3) + l2*qr1_dot*r3*sin(qq3) + l2*qr2_dot*r3*sin(qq3) - 2*l2*qr3_dot*r3*sin(qq3) - 5*l2*qr1_dot*r3*sin(2*qq1 + 2*qq2 + qq3) - 5*l2*qr2_dot*r3*sin(2*qq1 + 2*qq2 + qq3) - 2*l2*qr3_dot*r3*sin(2*qq1 + 2*qq2 + qq3),                                                                                                            qr1_ddot*r4 + qr2_ddot*r4 + qr3_ddot*r4 + qr4_ddot*r4 + l3*qr1_ddot*cos(qq4) + l3*qr2_ddot*cos(qq4) + l3*qr3_ddot*cos(qq4) + (l3*qr4_ddot*cos(qq4))/2 + qr1_ddot*r3*cos(qq4) + qr2_ddot*r3*cos(qq4) + qr3_ddot*r3*cos(qq4) + (qr4_ddot*r3*cos(qq4))/2 + l3*qr1_dot*sin(qq4) + l3*qr2_dot*sin(qq4) + l3*qr3_dot*sin(qq4) - 3*l3*qr4_dot*sin(qq4) + qr1_dot*r3*sin(qq4) + qr2_dot*r3*sin(qq4) + qr3_dot*r3*sin(qq4) - 3*qr4_dot*r3*sin(qq4) + l1*qr1_ddot*cos(qq2 + qq3 + qq4) - 2*l1*qr1_dot*sin(qq2 + qq3 + qq4) - 2*l1*qr2_dot*sin(qq2 + qq3 + qq4) - 2*l1*qr3_dot*sin(qq2 + qq3 + qq4) - 2*l1*qr4_dot*sin(qq2 + qq3 + qq4) + 2*l2*qr1_ddot*cos(qq3 + qq4) + 2*l2*qr2_ddot*cos(qq3 + qq4) + l2*qr3_ddot*cos(qq3 + qq4) + l2*qr4_ddot*cos(qq3 + qq4) - l3*qr1_ddot*cos(2*qq1 + 2*qq2 + 2*qq3 + qq4) - l3*qr2_ddot*cos(2*qq1 + 2*qq2 + 2*qq3 + qq4) - l3*qr3_ddot*cos(2*qq1 + 2*qq2 + 2*qq3 + qq4) - (l3*qr4_ddot*cos(2*qq1 + 2*qq2 + 2*qq3 + qq4))/2 + qr1_ddot*r3*cos(2*qq1 + 2*qq2 + 2*qq3 + qq4) + qr2_ddot*r3*cos(2*qq1 + 2*qq2 + 2*qq3 + qq4) + qr3_ddot*r3*cos(2*qq1 + 2*qq2 + 2*qq3 + qq4) + (qr4_ddot*r3*cos(2*qq1 + 2*qq2 + 2*qq3 + qq4))/2 + 4*l2*qr1_dot*sin(qq3 + qq4) + 4*l2*qr2_dot*sin(qq3 + qq4) - 4*l2*qr3_dot*sin(qq3 + qq4) - 4*l2*qr4_dot*sin(qq3 + qq4) + 7*l3*qr1_dot*sin(2*qq1 + 2*qq2 + 2*qq3 + qq4) + 7*l3*qr2_dot*sin(2*qq1 + 2*qq2 + 2*qq3 + qq4) + 7*l3*qr3_dot*sin(2*qq1 + 2*qq2 + 2*qq3 + qq4) + 3*l3*qr4_dot*sin(2*qq1 + 2*qq2 + 2*qq3 + qq4) - 7*qr1_dot*r3*sin(2*qq1 + 2*qq2 + 2*qq3 + qq4) - 7*qr2_dot*r3*sin(2*qq1 + 2*qq2 + 2*qq3 + qq4) - 7*qr3_dot*r3*sin(2*qq1 + 2*qq2 + 2*qq3 + qq4) - 3*qr4_dot*r3*sin(2*qq1 + 2*qq2 + 2*qq3 + qq4), 0, 0, 0, 0, 0; ...
    0,        0,                   0, qr1_ddot + qr2_ddot + qr3_ddot, qr1_ddot + qr2_ddot + qr3_ddot + qr4_ddot,             0,                                                                                                                         0, 0,                                                                                                                                                         0,                                                                                        qr1_ddot*r3 + qr2_ddot*r3 + qr3_ddot*r3 + l2*qr1_ddot*cos(qq3) + l2*qr2_ddot*cos(qq3) - 4*l2*qr1_dot*sin(qq3) - 4*l2*qr2_dot*sin(qq3) - 4*l2*qr3_dot*sin(qq3) + l1*qr1_ddot*cos(qq2 + qq3) - 2*l1*qr1_dot*sin(qq2 + qq3) - 2*l1*qr2_dot*sin(qq2 + qq3) - 2*l1*qr3_dot*sin(qq2 + qq3), 0,                                                                                                                                                                                                                                                                                                                                                                                                                                                                                                                                                                                                     (l3^2*qr1_ddot)/2 + (l3^2*qr2_ddot)/2 + (l3^2*qr3_ddot)/2 + (qr1_ddot*r3^2)/2 + (qr2_ddot*r3^2)/2 + (qr3_ddot*r3^2)/2 - (l3^2*qr1_ddot*cos(2*qq1 + 2*qq2 + 2*qq3))/2 - (l3^2*qr2_ddot*cos(2*qq1 + 2*qq2 + 2*qq3))/2 - (l3^2*qr3_ddot*cos(2*qq1 + 2*qq2 + 2*qq3))/2 + (qr1_ddot*r3^2*cos(2*qq1 + 2*qq2 + 2*qq3))/2 + (qr2_ddot*r3^2*cos(2*qq1 + 2*qq2 + 2*qq3))/2 + (qr3_ddot*r3^2*cos(2*qq1 + 2*qq2 + 2*qq3))/2 + 3*l3^2*qr1_dot*sin(2*qq1 + 2*qq2 + 2*qq3) + 3*l3^2*qr2_dot*sin(2*qq1 + 2*qq2 + 2*qq3) + 3*l3^2*qr3_dot*sin(2*qq1 + 2*qq2 + 2*qq3) - 3*qr1_dot*r3^2*sin(2*qq1 + 2*qq2 + 2*qq3) - 3*qr2_dot*r3^2*sin(2*qq1 + 2*qq2 + 2*qq3) - 3*qr3_dot*r3^2*sin(2*qq1 + 2*qq2 + 2*qq3) - (l1*l3*qr1_ddot*cos(2*qq1 + qq2 + qq3))/2 + (l1*qr1_ddot*r3*cos(2*qq1 + qq2 + qq3))/2 + l1*l3*qr1_dot*sin(2*qq1 + qq2 + qq3) + l1*l3*qr2_dot*sin(2*qq1 + qq2 + qq3) + l1*l3*qr3_dot*sin(2*qq1 + qq2 + qq3) - l1*qr1_dot*r3*sin(2*qq1 + qq2 + qq3) - l1*qr2_dot*r3*sin(2*qq1 + qq2 + qq3) - l1*qr3_dot*r3*sin(2*qq1 + qq2 + qq3) + (l1*l3*qr1_ddot*cos(qq2 + qq3))/2 + (l1*qr1_ddot*r3*cos(qq2 + qq3))/2 - l1*l3*qr1_dot*sin(qq2 + qq3) - l1*l3*qr2_dot*sin(qq2 + qq3) - l1*l3*qr3_dot*sin(qq2 + qq3) - l1*qr1_dot*r3*sin(qq2 + qq3) - l1*qr2_dot*r3*sin(qq2 + qq3) - l1*qr3_dot*r3*sin(qq2 + qq3) + (l2*l3*qr1_ddot*cos(qq3))/2 + (l2*l3*qr2_ddot*cos(qq3))/2 - (l2*l3*qr1_ddot*cos(2*qq1 + 2*qq2 + qq3))/2 - (l2*l3*qr2_ddot*cos(2*qq1 + 2*qq2 + qq3))/2 + (l2*qr1_ddot*r3*cos(qq3))/2 + (l2*qr2_ddot*r3*cos(qq3))/2 + (l2*qr1_ddot*r3*cos(2*qq1 + 2*qq2 + qq3))/2 + (l2*qr2_ddot*r3*cos(2*qq1 + 2*qq2 + qq3))/2 - 2*l2*l3*qr1_dot*sin(qq3) - 2*l2*l3*qr2_dot*sin(qq3) - 2*l2*l3*qr3_dot*sin(qq3) + 2*l2*l3*qr1_dot*sin(2*qq1 + 2*qq2 + qq3) + 2*l2*l3*qr2_dot*sin(2*qq1 + 2*qq2 + qq3) + 2*l2*l3*qr3_dot*sin(2*qq1 + 2*qq2 + qq3) - 2*l2*qr1_dot*r3*sin(qq3) - 2*l2*qr2_dot*r3*sin(qq3) - 2*l2*qr3_dot*r3*sin(qq3) - 2*l2*qr1_dot*r3*sin(2*qq1 + 2*qq2 + qq3) - 2*l2*qr2_dot*r3*sin(2*qq1 + 2*qq2 + qq3) - 2*l2*qr3_dot*r3*sin(2*qq1 + 2*qq2 + qq3),                                                                                                                                                                          qr1_ddot*r4 + qr2_ddot*r4 + qr3_ddot*r4 + qr4_ddot*r4 + l3*qr1_ddot*cos(qq4) + l3*qr2_ddot*cos(qq4) + l3*qr3_ddot*cos(qq4) + (l3*qr4_ddot*cos(qq4))/2 + qr1_ddot*r3*cos(qq4) + qr2_ddot*r3*cos(qq4) + qr3_ddot*r3*cos(qq4) + (qr4_ddot*r3*cos(qq4))/2 + l3*qr1_dot*sin(qq4) + l3*qr2_dot*sin(qq4) + l3*qr3_dot*sin(qq4) - 3*l3*qr4_dot*sin(qq4) + qr1_dot*r3*sin(qq4) + qr2_dot*r3*sin(qq4) + qr3_dot*r3*sin(qq4) - 3*qr4_dot*r3*sin(qq4) + l1*qr1_ddot*cos(qq2 + qq3 + qq4) - 2*l1*qr1_dot*sin(qq2 + qq3 + qq4) - 2*l1*qr2_dot*sin(qq2 + qq3 + qq4) - 2*l1*qr3_dot*sin(qq2 + qq3 + qq4) - 2*l1*qr4_dot*sin(qq2 + qq3 + qq4) + l2*qr1_ddot*cos(qq3 + qq4) + l2*qr2_ddot*cos(qq3 + qq4) - l3*qr1_ddot*cos(2*qq1 + 2*qq2 + 2*qq3 + qq4) - l3*qr2_ddot*cos(2*qq1 + 2*qq2 + 2*qq3 + qq4) - l3*qr3_ddot*cos(2*qq1 + 2*qq2 + 2*qq3 + qq4) - (l3*qr4_ddot*cos(2*qq1 + 2*qq2 + 2*qq3 + qq4))/2 + qr1_ddot*r3*cos(2*qq1 + 2*qq2 + 2*qq3 + qq4) + qr2_ddot*r3*cos(2*qq1 + 2*qq2 + 2*qq3 + qq4) + qr3_ddot*r3*cos(2*qq1 + 2*qq2 + 2*qq3 + qq4) + (qr4_ddot*r3*cos(2*qq1 + 2*qq2 + 2*qq3 + qq4))/2 - 4*l2*qr1_dot*sin(qq3 + qq4) - 4*l2*qr2_dot*sin(qq3 + qq4) - 4*l2*qr3_dot*sin(qq3 + qq4) - 4*l2*qr4_dot*sin(qq3 + qq4) + 7*l3*qr1_dot*sin(2*qq1 + 2*qq2 + 2*qq3 + qq4) + 7*l3*qr2_dot*sin(2*qq1 + 2*qq2 + 2*qq3 + qq4) + 7*l3*qr3_dot*sin(2*qq1 + 2*qq2 + 2*qq3 + qq4) + 3*l3*qr4_dot*sin(2*qq1 + 2*qq2 + 2*qq3 + qq4) - 7*qr1_dot*r3*sin(2*qq1 + 2*qq2 + 2*qq3 + qq4) - 7*qr2_dot*r3*sin(2*qq1 + 2*qq2 + 2*qq3 + qq4) - 7*qr3_dot*r3*sin(2*qq1 + 2*qq2 + 2*qq3 + qq4) - 3*qr4_dot*r3*sin(2*qq1 + 2*qq2 + 2*qq3 + qq4), 0, 0, 0, 0, 0; ...
    0,        0,                   0,                              0, qr1_ddot + qr2_ddot + qr3_ddot + qr4_ddot,             0,                                                                                                                         0, 0,                                                                                                                                                         0,                                                                                                                                                                                                                                                                                                                                                                           0, 0,                                                                                                                                                                                                                                                                                                                                                                                                                                                                                                                                                                                                                                                                                                                                                                                                                                                                                                                                                                                                                                                                                                                                                                                                                                                                                                                                                                                                                                                                                                                                                                                                                                                                                                                                                                                                                                                                                                                                                                                                                                                                                                                                                                                                                                                                                                                                                                                                                                                                                                                                                                                                                                                   0,                                                                                                                                                                                                                                                                          qr1_ddot*r4 + qr2_ddot*r4 + qr3_ddot*r4 + qr4_ddot*r4 + (l3*qr1_ddot*cos(qq4))/2 + (l3*qr2_ddot*cos(qq4))/2 + (l3*qr3_ddot*cos(qq4))/2 + (qr1_ddot*r3*cos(qq4))/2 + (qr2_ddot*r3*cos(qq4))/2 + (qr3_ddot*r3*cos(qq4))/2 - 3*l3*qr1_dot*sin(qq4) - 3*l3*qr2_dot*sin(qq4) - 3*l3*qr3_dot*sin(qq4) - 3*l3*qr4_dot*sin(qq4) - 3*qr1_dot*r3*sin(qq4) - 3*qr2_dot*r3*sin(qq4) - 3*qr3_dot*r3*sin(qq4) - 3*qr4_dot*r3*sin(qq4) + l1*qr1_ddot*cos(qq2 + qq3 + qq4) - 2*l1*qr1_dot*sin(qq2 + qq3 + qq4) - 2*l1*qr2_dot*sin(qq2 + qq3 + qq4) - 2*l1*qr3_dot*sin(qq2 + qq3 + qq4) - 2*l1*qr4_dot*sin(qq2 + qq3 + qq4) + l2*qr1_ddot*cos(qq3 + qq4) + l2*qr2_ddot*cos(qq3 + qq4) - (l3*qr1_ddot*cos(2*qq1 + 2*qq2 + 2*qq3 + qq4))/2 - (l3*qr2_ddot*cos(2*qq1 + 2*qq2 + 2*qq3 + qq4))/2 - (l3*qr3_ddot*cos(2*qq1 + 2*qq2 + 2*qq3 + qq4))/2 + (qr1_ddot*r3*cos(2*qq1 + 2*qq2 + 2*qq3 + qq4))/2 + (qr2_ddot*r3*cos(2*qq1 + 2*qq2 + 2*qq3 + qq4))/2 + (qr3_ddot*r3*cos(2*qq1 + 2*qq2 + 2*qq3 + qq4))/2 - 4*l2*qr1_dot*sin(qq3 + qq4) - 4*l2*qr2_dot*sin(qq3 + qq4) - 4*l2*qr3_dot*sin(qq3 + qq4) - 4*l2*qr4_dot*sin(qq3 + qq4) + 3*l3*qr1_dot*sin(2*qq1 + 2*qq2 + 2*qq3 + qq4) + 3*l3*qr2_dot*sin(2*qq1 + 2*qq2 + 2*qq3 + qq4) + 3*l3*qr3_dot*sin(2*qq1 + 2*qq2 + 2*qq3 + qq4) + 3*l3*qr4_dot*sin(2*qq1 + 2*qq2 + 2*qq3 + qq4) - 3*qr1_dot*r3*sin(2*qq1 + 2*qq2 + 2*qq3 + qq4) - 3*qr2_dot*r3*sin(2*qq1 + 2*qq2 + 2*qq3 + qq4) - 3*qr3_dot*r3*sin(2*qq1 + 2*qq2 + 2*qq3 + qq4) - 3*qr4_dot*r3*sin(2*qq1 + 2*qq2 + 2*qq3 + qq4), 0, 0, 0, 0, 0]

== matlab function adaptive_multi_task/MATLAB Function5 ==
  data: q_r_1_dot output; x_1r_dot input; J_1 input; N_1 output; eta output
function [q_r_1_dot, N_1, eta] = func_q_r_1_dot(x_1r_dot, J_1)

q_r_0_dot = zeros(4, 1);
N_0 = eye(4) % dimension 맞추기
% J_1 = 
J_1_bar = J_1 * N_0
N_1 = eye(4) - pinv(J_1_bar)*J_1_bar
eta = [1;0;0;0]

q_r_1_dot = q_r_0_dot + N_0 * pinv(J_1_bar) * (x_1r_dot - J_1*q_r_0_dot) + N_1*eta

== matlab function adaptive_multi_task/MATLAB Function6 ==
  data: q_r_2_dot output; q_r_1_dot input; x_2r_dot input; J_2 input; N_1 input; eta input; N_2 output
function [q_r_2_dot, N_2] = func_q_r_2_dot(q_r_1_dot, x_2r_dot, J_2, N_1, eta)

% N_0 = eye() % dimension 맞추기
% J_1 = 
% J_1_bar = J_1 * N_0
% N_1 = eye(4) - pinv(J_1_bar)*J_1_bar

% J_2 = 
J_2_bar = J_2 * N_1
N_2 = N_1 * (eye(4) - pinv(J_2_bar)*J_2_bar)
% eta = eye()

q_r_2_dot = q_r_1_dot + N_1 * pinv(J_2_bar) * (x_2r_dot - J_2*q_r_1_dot) + N_2*eta

== matlab function adaptive_multi_task/MATLAB Function7 ==
  data: q_r_3_dot output; q_r_2_dot input; x_3r_dot input; N_2 input; J_3 input; eta input
function q_r_3_dot = func_q_r_3_dot(q_r_2_dot, x_3r_dot, N_2, J_3, eta)

% N_0 = eye() % dimension 맞추기
% J_1 = 
% J_1_bar = J_1 * N_0
% N_1 = eye() - pinv(J_1_bar)*J_1_bar
% 
% J_2 = 
% J_2_bar = J_2 * N_1
% N_2 = N_1 * (eye() - pinv(J_2_bar)*J_2_bar)

% J_3 = 
J_3_bar = J_3 * N_2
N_3 = N_2 * (eye(4) - pinv(J_3_bar)*J_3_bar)
% eta = eye()

q_r_3_dot = q_r_2_dot + N_2 * pinv(J_3_bar) * (x_3r_dot - J_3*q_r_2_dot) + N_3*eta

== matlab function adaptive_multi_task/MATLAB Function8 ==
  data: x_1r_dot output; x_1d input; x_1d_dot input; x_1 input
function x_1r_dot = func_x_1r_dot(x_1d, x_1d_dot, x_1)

Gamma_1 = 5*eye(2)

x_1r_dot = x_1d_dot + Gamma_1*(x_1d - x_1)

== matlab function adaptive_multi_task/MATLAB Function9 ==
  data: x_1d output; t input; x_1d_dot output
function [x_1d, x_1d_dot] = func_x_1d(t)

x_1d = [sin(0.25*t)+0.2; cos(0.25*t)+0.15]
x_1d_dot = [0.25*cos(0.25*t); -0.25*sin(0.25*t)]

== matlab function adaptive_multi_task/MATLAB Function10 ==
  data: x_1d input; x output; y output
function [x, y] = fcn(x_1d)


x = x_1d(1)
y = x_1d(2)
